simulink model "gm_Transformation_V12"  (R2022a)
settings: Solver=FixedStepDiscrete  StartTime=0.0  StopTime=10.0  RelTol=1e-3
InitFcn:
  | Ts_xadc = 0.1;
undefined symbols (not defined in the file or in its folder): T_25MHz, T_mech
libraries: hdlsllib x14, simulink x13, hdlmdlgenlib x6, simulink_need_slupdate x1
(part 2 of 4)

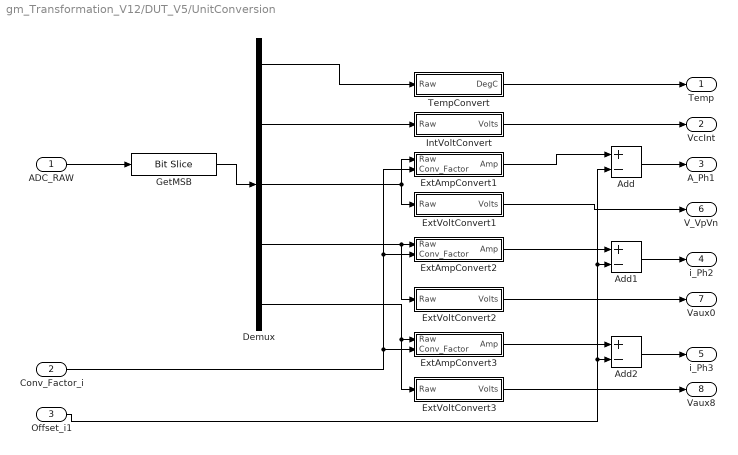
== system gm_Transformation_V12/DUT_V5/UnitConversion ==
  ADC_RAW : Inport
  Conv_Factor_i : Inport  Port=2
  Offset_i1 : Inport  Port=3
  Add : Sum  Inputs=+-  OutDataTypeStr=fixdt(1,16,11)
  Add1 : Sum  Inputs=+-  OutDataTypeStr=fixdt(1,16,11)
  Add2 : Sum  Inputs=+-  OutDataTypeStr=fixdt(1,16,11)
  Demux : Demux  Outputs=5
  ExtAmpConvert1 : Subsystem  TreatAsAtomicUnit=on
  ExtAmpConvert2 : Subsystem  TreatAsAtomicUnit=on
  ExtAmpConvert3 : Subsystem  TreatAsAtomicUnit=on
  ExtVoltConvert1 : Subsystem  TreatAsAtomicUnit=on
  ExtVoltConvert2 : Subsystem  TreatAsAtomicUnit=on
  ExtVoltConvert3 : Subsystem  TreatAsAtomicUnit=on
  GetMSB : hdlsllib/Logic and Bit Operations/Bit Slice  lidx=15  ridx=4
      settings: SourceProductBaseCode=SL
  IntVoltConvert : Subsystem  TreatAsAtomicUnit=on
  TempConvert : Subsystem
  Temp : Outport  VectorParamsAs1DForOutWhenUnconnected=off
  VccInt : Outport  Port=2  VectorParamsAs1DForOutWhenUnconnected=off
  A_Ph1 : Outport  Port=3  VectorParamsAs1DForOutWhenUnconnected=off
  i_Ph2 : Outport  Port=4  VectorParamsAs1DForOutWhenUnconnected=off
  i_Ph3 : Outport  Port=5  VectorParamsAs1DForOutWhenUnconnected=off
  V_VpVn : Outport  Port=6  VectorParamsAs1DForOutWhenUnconnected=off
  Vaux0 : Outport  Port=7  VectorParamsAs1DForOutWhenUnconnected=off
  Vaux8 : Outport  Port=8  VectorParamsAs1DForOutWhenUnconnected=off
  wires:
  Offset_i1/1 -> Add1/2, Add/2, Add2/2
  Add2/1 -> i_Ph3/1
  ExtAmpConvert3/1(Amp) -> Add2/1
  Add1/1 -> i_Ph2/1
  ExtAmpConvert2/1(Amp) -> Add1/1
  Add/1 -> A_Ph1/1
  ExtVoltConvert1/1(Volts) -> V_VpVn/1
  Conv_Factor_i/1 -> ExtAmpConvert1/2(Conv_Factor), ExtAmpConvert2/2(Conv_Factor), ExtAmpConvert3/2(Conv_Factor)
  Demux/5 -> ExtVoltConvert3/1(Raw), ExtAmpConvert3/1(Raw)
  Demux/4 -> ExtAmpConvert2/1(Raw), ExtVoltConvert2/1(Raw)
  Demux/3 -> ExtAmpConvert1/1(Raw), ExtVoltConvert1/1(Raw)
  Demux/2 -> IntVoltConvert/1(Raw)
  Demux/1 -> TempConvert/1(Raw)
  ExtVoltConvert3/1(Volts) -> Vaux8/1
  ExtVoltConvert2/1(Volts) -> Vaux0/1
  ExtAmpConvert1/1(Amp) -> Add/1
  IntVoltConvert/1(Volts) -> VccInt/1
  TempConvert/1(DegC) -> Temp/1
  GetMSB/1 -> Demux/1
  ADC_RAW/1 -> GetMSB/1

== system gm_Transformation_V12/Trans_123_dq_fix_V12/Delay10_controlled ==
  in0 : Inport  OutDataTypeStr=fixdt(1, 18, 11)  SampleTime=4e-08
  stateControl : EnablePort  OutDataTypeStr=boolean
  Delay10 : Delay  DelayLength=double(1)  InitialCondition=0  SampleTime=4e-08
  out0 : Outport  OutDataTypeStr=fixdt(1, 18, 11)  SampleTime=4e-08
  wires:
  Delay10/1 -> out0/1
  in0/1 -> Delay10/1

== system gm_Transformation_V12/Trans_123_dq_fix_V12/Delay16_controlled ==
  in0 : Inport  OutDataTypeStr=fixdt(1, 18, 11)  SampleTime=4e-08
  stateControl : EnablePort  OutDataTypeStr=boolean
  Delay16 : Delay  DelayLength=double(1)  InitialCondition=0  SampleTime=4e-08
  out0 : Outport  OutDataTypeStr=fixdt(1, 18, 11)  SampleTime=4e-08
  wires:
  Delay16/1 -> out0/1
  in0/1 -> Delay16/1

== system gm_Transformation_V12/Trans_123_dq_fix_V12/Delay1_controlled ==
  in0 : Inport  OutDataTypeStr=fixdt(1, 18, 11)  SampleTime=4e-08
  stateControl : EnablePort  OutDataTypeStr=boolean
  Delay1 : Delay  DelayLength=double(1)  InitialCondition=0  SampleTime=4e-08
  out0 : Outport  OutDataTypeStr=fixdt(1, 18, 11)  SampleTime=4e-08
  wires:
  Delay1/1 -> out0/1
  in0/1 -> Delay1/1

== system gm_Transformation_V12/Trans_123_dq_fix_V12/Delay22_controlled ==
  in0 : Inport  OutDataTypeStr=fixdt(1, 18, 11)  SampleTime=4e-08
  stateControl : EnablePort  OutDataTypeStr=boolean
  Delay22 : Delay  DelayLength=double(1)  InitialCondition=0  SampleTime=4e-08
  out0 : Outport  OutDataTypeStr=fixdt(1, 18, 11)  SampleTime=4e-08
  wires:
  Delay22/1 -> out0/1
  in0/1 -> Delay22/1

== system gm_Transformation_V12/Trans_123_dq_fix_V12/Delay2_controlled ==
  in0 : Inport  OutDataTypeStr=fixdt(1, 18, 11)  SampleTime=4e-08
  stateControl : EnablePort  OutDataTypeStr=boolean
  Delay2 : Delay  DelayLength=double(1)  InitialCondition=0  SampleTime=4e-08
  out0 : Outport  OutDataTypeStr=fixdt(1, 18, 11)  SampleTime=4e-08
  wires:
  Delay2/1 -> out0/1
  in0/1 -> Delay2/1

== system gm_Transformation_V12/Trans_123_dq_fix_V12/Delay3_controlled ==
  in0 : Inport  OutDataTypeStr=fixdt(1, 16, 14)  SampleTime=4e-08
  stateControl : EnablePort  OutDataTypeStr=boolean
  Delay3 : Delay  DelayLength=double(1)  InitialCondition=0  SampleTime=4e-08
  out0 : Outport  OutDataTypeStr=fixdt(1, 16, 14)  SampleTime=4e-08
  wires:
  Delay3/1 -> out0/1
  in0/1 -> Delay3/1

== system gm_Transformation_V12/Trans_123_dq_fix_V12/Delay4_controlled ==
  in0 : Inport  OutDataTypeStr=fixdt(1, 18, 11)  SampleTime=4e-08
  stateControl : EnablePort  OutDataTypeStr=boolean
  Delay4 : Delay  DelayLength=double(1)  InitialCondition=0  SampleTime=4e-08
  out0 : Outport  OutDataTypeStr=fixdt(1, 18, 11)  SampleTime=4e-08
  wires:
  Delay4/1 -> out0/1
  in0/1 -> Delay4/1

== system gm_Transformation_V12/Trans_123_dq_fix_V12/Delay5_controlled ==
  in0 : Inport  OutDataTypeStr=fixdt(1, 18, 11)  SampleTime=4e-08
  stateControl : EnablePort  OutDataTypeStr=boolean
  Delay5 : Delay  DelayLength=double(1)  InitialCondition=0  SampleTime=4e-08
  out0 : Outport  OutDataTypeStr=fixdt(1, 18, 11)  SampleTime=4e-08
  wires:
  Delay5/1 -> out0/1
  in0/1 -> Delay5/1

== system gm_Transformation_V12/Trans_123_dq_fix_V12/Delay7_controlled ==
  in0 : Inport  OutDataTypeStr=fixdt(1, 16, 14)  SampleTime=4e-08
  stateControl : EnablePort  OutDataTypeStr=boolean
  Delay7 : Delay  DelayLength=double(1)  InitialCondition=0  SampleTime=4e-08
  out0 : Outport  OutDataTypeStr=fixdt(1, 16, 14)  SampleTime=4e-08
  wires:
  Delay7/1 -> out0/1
  in0/1 -> Delay7/1

== system gm_Transformation_V12/Trans_123_dq_fix_V12/reset_old2_controlled ==
  in0 : Inport  OutDataTypeStr=boolean  SampleTime=4e-08
  stateControl : EnablePort  OutDataTypeStr=boolean
  reset_old2 : Delay  DelayLength=double(1)  InitialCondition=0  SampleTime=4e-08
  out0 : Outport  OutDataTypeStr=boolean  SampleTime=4e-08
  wires:
  reset_old2/1 -> out0/1
  in0/1 -> reset_old2/1

== system gm_Transformation_V12/xadc/xadc_plant ==
  Addr : Inport
  V : Inport  Port=2
  Vaux : Inport  Port=3
  AuxChan : Subsystem
  Bit Slice : hdlsllib/Logic and Bit Operations/Bit Slice  lidx=3  ridx=0
      settings: SourceProductBaseCode=SL
  Bit Slice1 : hdlsllib/Logic and Bit Operations/Bit Slice  lidx=4  ridx=4
      settings: SourceProductBaseCode=SL
  IntChan : Subsystem
  Switch : Switch  Criteria=u2 ~= 0  SaturateOnIntegerOverflow=off  InputSameDT=off
  Data : Outport  VectorParamsAs1DForOutWhenUnconnected=off
  wires:
  AuxChan/1(Aux_ADC) -> Switch/1
  IntChan/1(Int_ADC) -> Switch/3
  Bit Slice1/1 -> Switch/2
  Switch/1 -> Data/1
  V/1 -> IntChan/2(V)
  Vaux/1 -> AuxChan/2(Vaux)
  Bit Slice/1 -> AuxChan/1(Addr), IntChan/1(Addr)
  Addr/1 -> Bit Slice/1, Bit Slice1/1

== system gm_Transformation_V12/DUT_V5/UnitConversion/ExtAmpConvert1 ==
  Raw : Inport
  Conv_Factor : Inport  Port=2
  Product : Product  OutDataTypeStr=fixdt(1,16,11)
  Amp : Outport  VectorParamsAs1DForOutWhenUnconnected=off
  wires:
  Conv_Factor/1 -> Product/2
  Product/1 -> Amp/1
  Raw/1 -> Product/1

== system gm_Transformation_V12/DUT_V5/UnitConversion/ExtAmpConvert2 ==
  Raw : Inport
  Conv_Factor : Inport  Port=2
  Product : Product  OutDataTypeStr=fixdt(1,16,11)
  Amp : Outport  VectorParamsAs1DForOutWhenUnconnected=off
  wires:
  Conv_Factor/1 -> Product/2
  Product/1 -> Amp/1
  Raw/1 -> Product/1

== system gm_Transformation_V12/DUT_V5/UnitConversion/ExtAmpConvert3 ==
  Raw : Inport
  Conv_Factor : Inport  Port=2
  Product : Product  OutDataTypeStr=fixdt(1,16,11)
  Amp : Outport  VectorParamsAs1DForOutWhenUnconnected=off
  wires:
  Conv_Factor/1 -> Product/2
  Product/1 -> Amp/1
  Raw/1 -> Product/1

== system gm_Transformation_V12/DUT_V5/UnitConversion/ExtVoltConvert1 ==
  Raw : Inport
  Gain : Gain  Gain=fi(1/4096)  OutMin=0  OutMax=1  OutDataTypeStr=fixdt(0,16)
  Volts : Outport  VectorParamsAs1DForOutWhenUnconnected=off
  wires:
  Gain/1 -> Volts/1
  Raw/1 -> Gain/1

== system gm_Transformation_V12/DUT_V5/UnitConversion/ExtVoltConvert2 ==
  Raw : Inport
  Gain : Gain  Gain=fi(1/4096)  OutMin=0  OutMax=1  OutDataTypeStr=fixdt(0,16)
  Volts : Outport  VectorParamsAs1DForOutWhenUnconnected=off
  wires:
  Raw/1 -> Gain/1
  Gain/1 -> Volts/1

== system gm_Transformation_V12/DUT_V5/UnitConversion/ExtVoltConvert3 ==
  Raw : Inport
  Gain : Gain  Gain=fi(1/4096)  OutMin=0  OutMax=1  OutDataTypeStr=fixdt(0,16)
  Volts : Outport  VectorParamsAs1DForOutWhenUnconnected=off
  wires:
  Gain/1 -> Volts/1
  Raw/1 -> Gain/1

== system gm_Transformation_V12/DUT_V5/UnitConversion/IntVoltConvert ==
  Raw : Inport
  Gain : Gain  Gain=fi(3/4096)  OutMin=0  OutMax=3  OutDataTypeStr=fixdt(0,16)
  Volts : Outport  VectorParamsAs1DForOutWhenUnconnected=off
  wires:
  Gain/1 -> Volts/1
  Raw/1 -> Gain/1

== system gm_Transformation_V12/DUT_V5/UnitConversion/TempConvert ==
  Raw : Inport
  Add : Sum  Inputs=+-
  Constant : Constant  Value=273.15  OutDataTypeStr=fixdt(0,15)  SampleTime=-1
  Gain : Gain  Gain=fi(503.975/4096)  OutMin=0  OutMax=503.975  OutDataTypeStr=fixdt(0,15)
  DegC : Outport  VectorParamsAs1DForOutWhenUnconnected=off
  wires:
  Raw/1 -> Gain/1
  Add/1 -> DegC/1
  Constant/1 -> Add/2
  Gain/1 -> Add/1

== system gm_Transformation_V12/xadc/xadc_plant/AuxChan ==
  Addr : Inport
  Vaux : Inport  Port=2
  Demux : Demux  Outputs=16
  ExtVoltPlant19 : Subsystem
  Multiport Switch1 : MultiPortSwitch  DataPortOrder=Zero-based contiguous  Inputs=16  DiagnosticForDefault=None  zeroidx=on  SaturateOnIntegerOverflow=off  InputSameDT=off
  Aux_ADC : Outport  VectorParamsAs1DForOutWhenUnconnected=off
  wires:
  Demux/16 -> Multiport Switch1/17
  Addr/1 -> Multiport Switch1/1
  Demux/15 -> Multiport Switch1/16
  Multiport Switch1/1 -> Aux_ADC/1
  Demux/9 -> Multiport Switch1/10
  Vaux/1 -> ExtVoltPlant19/1(Volts)
  Demux/7 -> Multiport Switch1/8
  Demux/5 -> Multiport Switch1/6
  Demux/13 -> Multiport Switch1/14
  Demux/11 -> Multiport Switch1/12
  Demux/10 -> Multiport Switch1/11
  Demux/4 -> Multiport Switch1/5
  Demux/14 -> Multiport Switch1/15
  Demux/6 -> Multiport Switch1/7
  Demux/12 -> Multiport Switch1/13
  Demux/8 -> Multiport Switch1/9
  Demux/2 -> Multiport Switch1/3
  Demux/3 -> Multiport Switch1/4
  Demux/1 -> Multiport Switch1/2
  ExtVoltPlant19/1(Raw_ADC) -> Demux/1

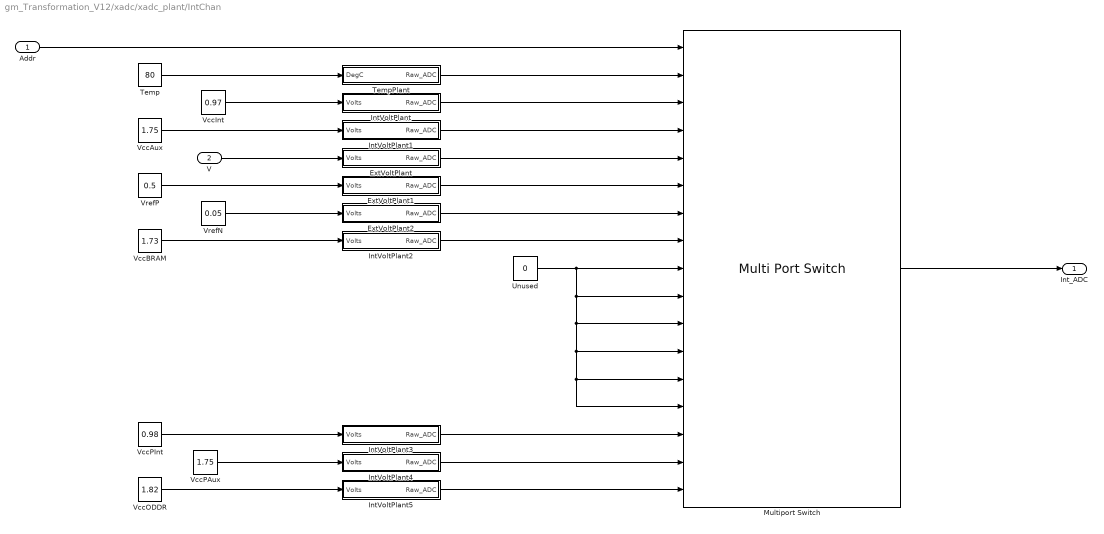
== system gm_Transformation_V12/xadc/xadc_plant/IntChan ==
  Addr : Inport
  V : Inport  Port=2
  ExtVoltPlant : Subsystem
  ExtVoltPlant1 : Subsystem
  ExtVoltPlant2 : Subsystem
  IntVoltPlant : Subsystem
  IntVoltPlant1 : Subsystem
  IntVoltPlant2 : Subsystem
  IntVoltPlant3 : Subsystem
  IntVoltPlant4 : Subsystem
  IntVoltPlant5 : Subsystem
  Multiport Switch : MultiPortSwitch  DataPortOrder=Zero-based contiguous  Inputs=16  DiagnosticForDefault=None  zeroidx=on  SaturateOnIntegerOverflow=off  InputSameDT=off
  Temp : Constant  Value=80  SampleTime=-1
  TempPlant : Subsystem
  Unused : Constant  Value=0  OutDataTypeStr=Inherit: Inherit via back propagation  SampleTime=-1
  VccAux : Constant  Value=1.75  SampleTime=-1
  VccBRAM : Constant  Value=1.73  SampleTime=-1
  VccInt : Constant  Value=0.97  SampleTime=-1
  VccODDR : Constant  Value=1.82  SampleTime=-1
  VccPAux : Constant  Value=1.75  SampleTime=-1
  VccPInt : Constant  Value=0.98  SampleTime=-1
  VrefN : Constant  Value=0.05  SampleTime=-1
  VrefP : Constant  Value=0.5  SampleTime=-1
  Int_ADC : Outport  VectorParamsAs1DForOutWhenUnconnected=off
  wires:
  VrefP/1 -> ExtVoltPlant1/1(Volts)
  ExtVoltPlant1/1(Raw_ADC) -> Multiport Switch/6
  IntVoltPlant1/1(Raw_ADC) -> Multiport Switch/4
  Unused/1 -> Multiport Switch/10, Multiport Switch/11, Multiport Switch/12, Multiport Switch/13, Multiport Switch/14, Multiport Switch/9
  IntVoltPlant/1(Raw_ADC) -> Multiport Switch/3
  Multiport Switch/1 -> Int_ADC/1
  Addr/1 -> Multiport Switch/1
  IntVoltPlant3/1(Raw_ADC) -> Multiport Switch/15
  VccBRAM/1 -> IntVoltPlant2/1(Volts)
  VccAux/1 -> IntVoltPlant1/1(Volts)
  VccPInt/1 -> IntVoltPlant3/1(Volts)
  VccPAux/1 -> IntVoltPlant4/1(Volts)
  ExtVoltPlant/1(Raw_ADC) -> Multiport Switch/5
  Temp/1 -> TempPlant/1(DegC)
  IntVoltPlant4/1(Raw_ADC) -> Multiport Switch/16
  VccInt/1 -> IntVoltPlant/1(Volts)
  TempPlant/1(Raw_ADC) -> Multiport Switch/2
  ExtVoltPlant2/1(Raw_ADC) -> Multiport Switch/7
  V/1 -> ExtVoltPlant/1(Volts)
  IntVoltPlant5/1(Raw_ADC) -> Multiport Switch/17
  VrefN/1 -> ExtVoltPlant2/1(Volts)
  VccODDR/1 -> IntVoltPlant5/1(Volts)
  IntVoltPlant2/1(Raw_ADC) -> Multiport Switch/8

== system gm_Transformation_V12/xadc/xadc_plant/AuxChan/ExtVoltPlant19 ==
  Volts : Inport
  Bit Concat : hdlsllib/Logic and Bit Operations/Bit Concat  numInputs=2
  Data Type Conversion : DataTypeConversion  OutDataTypeStr=fixdt(0,12,0)  SaturateOnIntegerOverflow=off  RndMeth=Floor
  Gain : Gain  Gain=4096
  LSB : Constant  Value=fi(0,0,4,0)  SampleTime=-1
  Raw_ADC : Outport  VectorParamsAs1DForOutWhenUnconnected=off
  wires:
  Gain/1 -> Data Type Conversion/1
  Volts/1 -> Gain/1
  Data Type Conversion/1 -> Bit Concat/1
  LSB/1 -> Bit Concat/2
  Bit Concat/1 -> Raw_ADC/1

== system gm_Transformation_V12/xadc/xadc_plant/IntChan/ExtVoltPlant ==
  Volts : Inport
  Bit Concat : hdlsllib/Logic and Bit Operations/Bit Concat  numInputs=2
  Data Type Conversion : DataTypeConversion  OutDataTypeStr=fixdt(0,12,0)  SaturateOnIntegerOverflow=off  RndMeth=Floor
  Gain : Gain  Gain=4096
  LSB : Constant  Value=fi(0,0,4,0)  SampleTime=-1
  Raw_ADC : Outport  VectorParamsAs1DForOutWhenUnconnected=off
  wires:
  Gain/1 -> Data Type Conversion/1
  Volts/1 -> Gain/1
  Data Type Conversion/1 -> Bit Concat/1
  LSB/1 -> Bit Concat/2
  Bit Concat/1 -> Raw_ADC/1

== system gm_Transformation_V12/xadc/xadc_plant/IntChan/ExtVoltPlant1 ==
  Volts : Inport
  Bit Concat : hdlsllib/Logic and Bit Operations/Bit Concat  numInputs=2
  Data Type Conversion : DataTypeConversion  OutDataTypeStr=fixdt(0,12,0)  SaturateOnIntegerOverflow=off  RndMeth=Floor
  Gain : Gain  Gain=4096
  LSB : Constant  Value=fi(0,0,4,0)  SampleTime=-1
  Raw_ADC : Outport  VectorParamsAs1DForOutWhenUnconnected=off
  wires:
  Bit Concat/1 -> Raw_ADC/1
  LSB/1 -> Bit Concat/2
  Data Type Conversion/1 -> Bit Concat/1
  Volts/1 -> Gain/1
  Gain/1 -> Data Type Conversion/1

== system gm_Transformation_V12/xadc/xadc_plant/IntChan/ExtVoltPlant2 ==
  Volts : Inport
  Bit Concat : hdlsllib/Logic and Bit Operations/Bit Concat  numInputs=2
  Data Type Conversion : DataTypeConversion  OutDataTypeStr=fixdt(0,12,0)  SaturateOnIntegerOverflow=off  RndMeth=Floor
  Gain : Gain  Gain=4096
  LSB : Constant  Value=fi(0,0,4,0)  SampleTime=-1
  Raw_ADC : Outport  VectorParamsAs1DForOutWhenUnconnected=off
  wires:
  Gain/1 -> Data Type Conversion/1
  Volts/1 -> Gain/1
  Data Type Conversion/1 -> Bit Concat/1
  LSB/1 -> Bit Concat/2
  Bit Concat/1 -> Raw_ADC/1

== system gm_Transformation_V12/xadc/xadc_plant/IntChan/IntVoltPlant ==
  Volts : Inport
  Bit Concat : hdlsllib/Logic and Bit Operations/Bit Concat  numInputs=2
  Data Type Conversion : DataTypeConversion  OutDataTypeStr=fixdt(0,12,0)  SaturateOnIntegerOverflow=off  RndMeth=Floor
  Gain : Gain  Gain=4096/3
  LSB : Constant  Value=fi(0,0,4,0)  SampleTime=-1
  Raw_ADC : Outport  VectorParamsAs1DForOutWhenUnconnected=off
  wires:
  Bit Concat/1 -> Raw_ADC/1
  LSB/1 -> Bit Concat/2
  Data Type Conversion/1 -> Bit Concat/1
  Volts/1 -> Gain/1
  Gain/1 -> Data Type Conversion/1

== system gm_Transformation_V12/xadc/xadc_plant/IntChan/IntVoltPlant1 ==
  Volts : Inport
  Bit Concat : hdlsllib/Logic and Bit Operations/Bit Concat  numInputs=2
  Data Type Conversion : DataTypeConversion  OutDataTypeStr=fixdt(0,12,0)  SaturateOnIntegerOverflow=off  RndMeth=Floor
  Gain : Gain  Gain=4096/3
  LSB : Constant  Value=fi(0,0,4,0)  SampleTime=-1
  Raw_ADC : Outport  VectorParamsAs1DForOutWhenUnconnected=off
  wires:
  Gain/1 -> Data Type Conversion/1
  Volts/1 -> Gain/1
  Data Type Conversion/1 -> Bit Concat/1
  LSB/1 -> Bit Concat/2
  Bit Concat/1 -> Raw_ADC/1

== system gm_Transformation_V12/xadc/xadc_plant/IntChan/IntVoltPlant2 ==
  Volts : Inport
  Bit Concat : hdlsllib/Logic and Bit Operations/Bit Concat  numInputs=2
  Data Type Conversion : DataTypeConversion  OutDataTypeStr=fixdt(0,12,0)  SaturateOnIntegerOverflow=off  RndMeth=Floor
  Gain : Gain  Gain=4096/3
  LSB : Constant  Value=fi(0,0,4,0)  SampleTime=-1
  Raw_ADC : Outport  VectorParamsAs1DForOutWhenUnconnected=off
  wires:
  Bit Concat/1 -> Raw_ADC/1
  LSB/1 -> Bit Concat/2
  Data Type Conversion/1 -> Bit Concat/1
  Volts/1 -> Gain/1
  Gain/1 -> Data Type Conversion/1

== system gm_Transformation_V12/xadc/xadc_plant/IntChan/IntVoltPlant3 ==
  Volts : Inport
  Bit Concat : hdlsllib/Logic and Bit Operations/Bit Concat  numInputs=2
  Data Type Conversion : DataTypeConversion  OutDataTypeStr=fixdt(0,12,0)  SaturateOnIntegerOverflow=off  RndMeth=Floor
  Gain : Gain  Gain=4096/3
  LSB : Constant  Value=fi(0,0,4,0)  SampleTime=-1
  Raw_ADC : Outport  VectorParamsAs1DForOutWhenUnconnected=off
  wires:
  Gain/1 -> Data Type Conversion/1
  Volts/1 -> Gain/1
  Data Type Conversion/1 -> Bit Concat/1
  LSB/1 -> Bit Concat/2
  Bit Concat/1 -> Raw_ADC/1

== system gm_Transformation_V12/xadc/xadc_plant/IntChan/IntVoltPlant4 ==
  Volts : Inport
  Bit Concat : hdlsllib/Logic and Bit Operations/Bit Concat  numInputs=2
  Data Type Conversion : DataTypeConversion  OutDataTypeStr=fixdt(0,12,0)  SaturateOnIntegerOverflow=off  RndMeth=Floor
  Gain : Gain  Gain=4096/3
  LSB : Constant  Value=fi(0,0,4,0)  SampleTime=-1
  Raw_ADC : Outport  VectorParamsAs1DForOutWhenUnconnected=off
  wires:
  Bit Concat/1 -> Raw_ADC/1
  LSB/1 -> Bit Concat/2
  Data Type Conversion/1 -> Bit Concat/1
  Volts/1 -> Gain/1
  Gain/1 -> Data Type Conversion/1

== system gm_Transformation_V12/xadc/xadc_plant/IntChan/IntVoltPlant5 ==
  Volts : Inport
  Bit Concat : hdlsllib/Logic and Bit Operations/Bit Concat  numInputs=2
  Data Type Conversion : DataTypeConversion  OutDataTypeStr=fixdt(0,12,0)  SaturateOnIntegerOverflow=off  RndMeth=Floor
  Gain : Gain  Gain=4096/3
  LSB : Constant  Value=fi(0,0,4,0)  SampleTime=-1
  Raw_ADC : Outport  VectorParamsAs1DForOutWhenUnconnected=off
  wires:
  Gain/1 -> Data Type Conversion/1
  Volts/1 -> Gain/1
  Data Type Conversion/1 -> Bit Concat/1
  LSB/1 -> Bit Concat/2
  Bit Concat/1 -> Raw_ADC/1

== system gm_Transformation_V12/xadc/xadc_plant/IntChan/TempPlant ==
  DegC : Inport
  Add : Sum
  Bit Concat : hdlsllib/Logic and Bit Operations/Bit Concat  numInputs=2
  Data Type Conversion : DataTypeConversion  OutDataTypeStr=fixdt(0,12,0)  SaturateOnIntegerOverflow=off  RndMeth=Floor
  Gain : Gain  Gain=4096/503.975
  LSB : Constant  Value=fi(0,0,4,0)  SampleTime=-1
  Offset : Constant  Value=273.15  SampleTime=-1
  Raw_ADC : Outport  VectorParamsAs1DForOutWhenUnconnected=off
  wires:
  Bit Concat/1 -> Raw_ADC/1
  Gain/1 -> Data Type Conversion/1
  LSB/1 -> Bit Concat/2
  Data Type Conversion/1 -> Bit Concat/1
  Add/1 -> Gain/1
  DegC/1 -> Add/1
  Offset/1 -> Add/2

== matlab function gm_Transformation_V12/Trans_123_dq_fix_V3/dq_transformation ==
  data: a input; d output; b input; theta input; q output
% Author : Saeid Saeidi
% Modified: Sebastian Wendel
% EAL -TUM
% MATLAB Version : R2016a
function [d, q]= fcn(a,b, theta )
% Defining persistent variables
%In VHDL , persistent variables will appear as Signals
persistent i1
persistent i2
persistent i3
persistent i4
persistent i5
persistent i6
persistent i7
persistent i8
persistent i9
persistent i10
persistent i11
persistent i12
persistent i13
persistent i14
persistent i15
persistent i16
% %
persistent i1n
persistent i2n
persistent i3n
persistent i4n
persistent i5n
persistent i6n
persistent i7n
persistent i8n
persistent i9n
persistent i10n
persistent i11n
persistent i12n
persistent i13n
persistent i14n
persistent i15n
persistent i16n
% %
persistent a1
persistent a2
persistent a3
persistent a4
persistent a5
persistent a6
persistent a7
persistent a8
persistent a9
persistent a10
persistent a11
persistent a12
persistent a13
persistent a14
persistent a15
persistent a16
% %
persistent b1
persistent b2
persistent b3
persistent b4
persistent b5
persistent b6
persistent b7
persistent b8
persistent b9
persistent b10
persistent b11
persistent b12
persistent b13
persistent b14
persistent b15
persistent b16
% %
persistent beta1
persistent beta2
persistent beta3
persistent beta4
persistent beta5
persistent beta6
persistent beta7
persistent beta8
persistent beta9
persistent beta10
persistent beta11
persistent beta12
persistent beta13
persistent beta14
persistent beta15
% %
persistent a1n
persistent a2n
persistent a3n
persistent a4n
persistent a5n
persistent a6n
persistent a7n
persistent a8n
persistent a9n
persistent a10n
persistent a11n
persistent a12n
persistent a13n
persistent a14n
persistent a15n
persistent a16n
% %
persistent b1n
persistent b2n
persistent b3n
persistent b4n
persistent b5n
persistent b6n
persistent b7n
persistent b8n
persistent b9n
persistent b10n
persistent b11n
persistent b12n
persistent b13n
persistent b14n
persistent b15n
persistent b16n
% %
persistent beta1n
persistent beta2n
persistent beta3n
persistent beta4n
persistent beta5n
persistent beta6n
persistent beta7n
persistent beta8n
persistent beta9n
persistent beta10n
persistent beta11n
persistent beta12n
persistent beta13n
persistent beta14n
persistent beta15n
% %
% Initialization of Persistent Variables with the numeric type of the
% input variables "a" and "b"
% After generating VHDL this part will be located in the RESET
if isempty (a1)
a1 = fi (0, numerictype (a), hdlfimath );
a2 = fi (0, numerictype (a), hdlfimath );
a3 = fi (0, numerictype (a), hdlfimath );
a4 = fi (0, numerictype (a), hdlfimath );
a5 = fi (0, numerictype (a), hdlfimath );
a6 = fi (0, numerictype (a), hdlfimath );
a7 = fi (0, numerictype (a), hdlfimath );
a8 = fi (0, numerictype (a), hdlfimath );
a9 = fi (0, numerictype (a), hdlfimath );
a10 = fi (0, numerictype (a), hdlfimath );
a11 = fi (0, numerictype (a), hdlfimath );
a12 = fi (0, numerictype (a), hdlfimath );
a13 = fi (0, numerictype (a), hdlfimath );
a14 = fi (0, numerictype (a), hdlfimath );
a15 = fi (0, numerictype (a), hdlfimath );
a16 = fi (0, numerictype (a), hdlfimath );
% %
b1 = fi (0, numerictype (b), hdlfimath );
b2 = fi (0, numerictype (b), hdlfimath );
b3 = fi (0, numerictype (b), hdlfimath );
b4 = fi (0, numerictype (b), hdlfimath );
b5 = fi (0, numerictype (b), hdlfimath );
b6 = fi (0, numerictype (b), hdlfimath );
b7 = fi (0, numerictype (b), hdlfimath );
b8 = fi (0, numerictype (b), hdlfimath );
b9 = fi (0, numerictype (b), hdlfimath );
b10 = fi (0, numerictype (b), hdlfimath );
b11 = fi (0, numerictype (b), hdlfimath );
b12 = fi (0, numerictype (b), hdlfimath );
b13 = fi (0, numerictype (b), hdlfimath );
b14 = fi (0, numerictype (b), hdlfimath );
b15 = fi (0, numerictype (b), hdlfimath );
b16 = fi (0, numerictype (b), hdlfimath );
% %
beta1 = fi (0, numerictype ( theta ), hdlfimath );
beta2 = fi (0, numerictype ( theta ), hdlfimath );
beta3 = fi (0, numerictype ( theta ), hdlfimath );
beta4 = fi (0, numerictype ( theta ), hdlfimath );
beta5 = fi (0, numerictype ( theta ), hdlfimath );
beta6 = fi (0, numerictype ( theta ), hdlfimath );
beta7 = fi (0, numerictype ( theta ), hdlfimath );
beta8 = fi (0, numerictype ( theta ), hdlfimath );
beta9 = fi (0, numerictype ( theta ), hdlfimath );
beta10 = fi (0, numerictype ( theta ), hdlfimath );
beta11 = fi (0, numerictype ( theta ), hdlfimath );
beta12 = fi (0, numerictype ( theta ), hdlfimath );
beta13 = fi (0, numerictype ( theta ), hdlfimath );
beta14 = fi (0, numerictype ( theta ), hdlfimath );
beta15 = fi (0, numerictype ( theta ), hdlfimath );
% %
a1n = fi (0, numerictype (a), hdlfimath );
a2n = fi (0, numerictype (a), hdlfimath );
a3n = fi (0, numerictype (a), hdlfimath );
a4n = fi (0, numerictype (a), hdlfimath );
a5n = fi (0, numerictype (a), hdlfimath );
a6n = fi (0, numerictype (a), hdlfimath );
a7n = fi (0, numerictype (a), hdlfimath );
a8n = fi (0, numerictype (a), hdlfimath );
a9n = fi (0, numerictype (a), hdlfimath );
a10n = fi (0, numerictype (a), hdlfimath );
a11n = fi (0, numerictype (a), hdlfimath );
a12n = fi (0, numerictype (a), hdlfimath );
a13n = fi (0, numerictype (a), hdlfimath );
a14n = fi (0, numerictype (a), hdlfimath );
a15n = fi (0, numerictype (a), hdlfimath );
a16n = fi (0, numerictype (a), hdlfimath );
% %
b1n = fi (0, numerictype (b), hdlfimath );
b2n = fi (0, numerictype (b), hdlfimath );
b3n = fi (0, numerictype (b), hdlfimath );
b4n = fi (0, numerictype (b), hdlfimath );
b5n = fi (0, numerictype (b), hdlfimath );
b6n = fi (0, numerictype (b), hdlfimath );
b7n = fi (0, numerictype (b), hdlfimath );
b8n = fi (0, numerictype (b), hdlfimath );
b9n = fi (0, numerictype (b), hdlfimath );
b10n = fi (0, numerictype (b), hdlfimath );
b11n = fi (0, numerictype (b), hdlfimath );
b12n = fi (0, numerictype (b), hdlfimath );
b13n = fi (0, numerictype (b), hdlfimath );
b14n = fi (0, numerictype (b), hdlfimath );
b15n = fi (0, numerictype (b), hdlfimath );
b16n = fi (0, numerictype (b), hdlfimath );
% %
beta1n = fi (0, numerictype ( theta ), hdlfimath );
beta2n = fi (0, numerictype ( theta ), hdlfimath );
beta3n = fi (0, numerictype ( theta ), hdlfimath );
beta4n = fi (0, numerictype ( theta ), hdlfimath );
beta5n = fi (0, numerictype ( theta ), hdlfimath );
beta6n = fi (0, numerictype ( theta ), hdlfimath );
beta7n = fi (0, numerictype ( theta ), hdlfimath );
beta8n = fi (0, numerictype ( theta ), hdlfimath );
beta9n = fi (0, numerictype ( theta ), hdlfimath );
beta10n = fi (0, numerictype ( theta ), hdlfimath );
beta11n = fi (0, numerictype ( theta ), hdlfimath );
beta12n = fi (0, numerictype ( theta ), hdlfimath );
beta13n = fi (0, numerictype ( theta ), hdlfimath );
beta14n = fi (0, numerictype ( theta ), hdlfimath );
beta15n = fi (0, numerictype ( theta ), hdlfimath );
% %
i1n = ufi (0 ,1 ,0);
i2n = ufi (0 ,1 ,0);
i3n = ufi (0 ,1 ,0);
i4n = ufi (0 ,1 ,0);
i5n = ufi (0 ,1 ,0);
i6n = ufi (0 ,1 ,0);
i7n = ufi (0 ,1 ,0);
i8n = ufi (0 ,1 ,0);
i9n = ufi (0 ,1 ,0);
i10n = ufi (0 ,1 ,0);
i11n = ufi (0 ,1 ,0);
i12n = ufi (0 ,1 ,0);
i13n = ufi (0 ,1 ,0);
i14n = ufi (0 ,1 ,0);
i15n = ufi (0 ,1 ,0);
i16n = ufi (0 ,1 ,0);
% %
i1 = ufi (0 ,1 ,0);
i2 = ufi (0 ,1 ,0);
i3 = ufi (0 ,1 ,0);
i4 = ufi (0 ,1 ,0);
i5 = ufi (0 ,1 ,0);
i6 = ufi (0 ,1 ,0);
i7 = ufi (0 ,1 ,0);
i8 = ufi (0 ,1 ,0);
i9 = ufi (0 ,1 ,0);
i10 = ufi (0 ,1 ,0);
i11 = ufi (0 ,1 ,0);
i12 = ufi (0 ,1 ,0);
i13 = ufi (0 ,1 ,0);
i14 = ufi (0 ,1 ,0);
i15 = ufi (0 ,1 ,0);
i16 = ufi (0 ,1 ,0);
end
%-----------------------------------------------------------------------%

% Definition of Constant Values
p       = fi(pi , numerictype ( theta ), hdlfimath );
p2      = fi(pi /2, numerictype ( theta ), hdlfimath ); %1.570796
p2m     = fi(-pi /2, numerictype ( theta ), hdlfimath );
theta0  = fi(theta , numerictype ( theta ), hdlfimath );

% Determining section of the theta -> Check if theta is between -pi/2 and
% pi/2
% -- ------- # First pipeline stage
if( theta0 <= fi(p2m , numerictype ( theta ), hdlfimath ))
    beta1n = fi( theta0 + p, numerictype ( theta ), hdlfimath );
    i1n = ufi (0 ,1 ,0);
elseif ( theta0 >= fi(p2 , numerictype ( theta ), hdlfimath ))
    beta1n = fi( theta0 - p, numerictype ( theta ), hdlfimath );
    i1n = ufi (0 ,1 ,0);
else
    beta1n = theta0 ;
    i1n = ufi (1 ,1 ,0);
end
a1n = fi(a, numerictype (a), hdlfimath );
b1n = fi(b, numerictype (b), hdlfimath );

% -- ------- # Second pipeline stage 0.78539816339745 = pi/4
if( beta1 <fi (0, numerictype ( theta ), hdlfimath ))
    a2n = fi(a1 + b1 , numerictype (a), hdlfimath );
    b2n = fi(b1 - a1 , numerictype (b), hdlfimath );
    beta2n = fi( beta1 + fi (0.78539816339745 , numerictype ( theta ) ,...
    hdlfimath ), numerictype ( theta ), hdlfimath );
else
    a2n = fi(a1 - b1 , numerictype (a), hdlfimath );
    b2n = fi(b1 + a1 , numerictype (b), hdlfimath );
    beta2n = fi( beta1 - fi (0.78539816339745 , numerictype ( theta ) ,...
    hdlfimath ), numerictype ( theta ), hdlfimath );
end

% -- ------- # Third pipeline stage 0.46364760900081 = pi/8 ???
if(beta2 <fi (0, numerictype ( theta ), hdlfimath ))
    a3n = fi(a2 + bitsra (b2 ,1) , numerictype (b), hdlfimath );
    b3n = fi(b2 - bitsra (a2 ,1) , numerictype (a), hdlfimath );
    beta3n = fi( beta2 + fi (0.46364760900081 , numerictype ( theta ) ,...
    hdlfimath ), numerictype ( theta ), hdlfimath );
else
    a3n = fi(a2 - bitsra (b2 ,1) , numerictype (a), hdlfimath );
    b3n = fi(b2 + bitsra (a2 ,1) , numerictype (b), hdlfimath );
    beta3n = fi( beta2 - fi (0.46364760900081 , numerictype ( theta ) ,...
    hdlfimath ), numerictype ( theta ), hdlfimath );
end

% -- ------- # Fourth pipeline stage
if(beta3 <fi (0, numerictype ( theta ), hdlfimath ))
    a4n = fi(a3 + bitsra (b3 ,2) , numerictype (a), hdlfimath );
    b4n = fi(b3 - bitsra (a3 ,2) , numerictype (b), hdlfimath );
    beta4n = fi( beta3 + fi (0.24497866312686 , numerictype ( theta ) ,...
    hdlfimath ), numerictype ( theta ), hdlfimath );
else
    a4n = fi(a3 - bitsra (b3 ,2) , numerictype (a), hdlfimath );
    b4n = fi(b3 + bitsra (a3 ,2) , numerictype (b), hdlfimath );
    beta4n = fi( beta3 - fi (0.24497866312686 , numerictype ( theta ) ,...
    hdlfimath ), numerictype ( theta ), hdlfimath );
end

% -- ------- # Fifth pipeline stage
if(beta4 <fi (0, numerictype ( theta ), hdlfimath ))
    a5n = fi(a4 + bitsra (b4 ,3) , numerictype (a), hdlfimath );
    b5n = fi(b4 - bitsra (a4 ,3) , numerictype (b), hdlfimath );
    beta5n = fi( beta4 + fi (0.12435499454676 , numerictype ( theta ) ,...
    hdlfimath ), numerictype ( theta ), hdlfimath );
else
    a5n = fi(a4 - bitsra (b4 ,3) , numerictype (a), hdlfimath );
    b5n = fi(b4 + bitsra (a4 ,3) , numerictype (b), hdlfimath );
    beta5n = fi( beta4 - fi (0.12435499454676 , numerictype ( theta ) ,...
    hdlfimath ), numerictype ( theta ), hdlfimath );
end

% -- ------- # Sixth pipeline stage
if(beta5 <fi (0, numerictype ( theta ), hdlfimath ))
    a6n = fi(a5 + bitsra (b5 ,4) , numerictype (a), hdlfimath );
    b6n = fi(b5 - bitsra (a5 ,4) , numerictype (b), hdlfimath );
    beta6n = fi( beta5 + fi (0.06241880999596 , numerictype ( theta ) ,...
    hdlfimath ), numerictype ( theta ), hdlfimath );
else
    a6n = fi(a5 - bitsra (b5 ,4) , numerictype (a), hdlfimath );
    b6n = fi( b5 + bitsra (a5 ,4) , numerictype (b), hdlfimath );
    beta6n = fi( beta5 - fi (0.06241880999596 , numerictype ( theta ) ,...
    hdlfimath ), numerictype ( theta ), hdlfimath );
end

% -- ------- # Seventh pipeline stage
if(beta6 <fi (0, numerictype ( theta ), hdlfimath ))
    a7n = fi(a6 + bitsra (b6 ,5) , numerictype (a), hdlfimath );
    b7n = fi(b6 - bitsra (a6 ,5) , numerictype (b), hdlfimath );
    beta7n = fi( beta6 + fi (0.03123983343027 , numerictype ( theta ) ,...
    hdlfimath ), numerictype ( theta ), hdlfimath );
else
    a7n = fi(a6 - bitsra (b6 ,5) , numerictype (a), hdlfimath );
    b7n = fi(b6 + bitsra (a6 ,5) , numerictype (b), hdlfimath );
    beta7n = fi( beta6 - fi (0.03123983343027 , numerictype ( theta ) ,...
    hdlfimath ), numerictype ( theta ), hdlfimath );
end

% -- ------- # Eighth pipeline stage
if(beta7 <fi (0, numerictype ( theta ), hdlfimath ))
    a8n = fi(a7 + bitsra (b7 ,6) , numerictype (a), hdlfimath );
    b8n = fi(b7 - bitsra (a7 ,6) , numerictype (b), hdlfimath );
    beta8n = fi( beta7 + fi (0.01562372862048 , numerictype ( theta ) ,...
    hdlfimath ), numerictype ( theta ), hdlfimath );
else
    a8n = fi(a7 - bitsra (b7 ,6) , numerictype (a), hdlfimath );
    b8n = fi(b7 + bitsra (a7 ,6) , numerictype (b), hdlfimath );
    beta8n = fi( beta7 - fi (0.01562372862048 , numerictype ( theta ) ,...
    hdlfimath ), numerictype ( theta ), hdlfimath );
end

% -- ------- # Ninth pipeline stage
if(beta8 <fi (0, numerictype ( theta ), hdlfimath ))
    a9n = fi(a8 + bitsra (b8 ,7) , numerictype (a), hdlfimath );
    b9n = fi(b8 - bitsra (a8 ,7) , numerictype (b), hdlfimath );
    beta9n = fi( beta8 + fi( 0.00781234106010 , numerictype ( theta ) ,...
    hdlfimath ), numerictype ( theta ), hdlfimath );
else
    a9n = fi(a8 - bitsra (b8 ,7) , numerictype (a), hdlfimath );
    b9n = fi( b8 + bitsra (a8 ,7) , numerictype (b), hdlfimath );
    beta9n = fi( beta8 - fi( 0.00781234106010 , numerictype ( theta ) ,...
    hdlfimath ), numerictype ( theta ), hdlfimath );
end

% -- ------- # Tenth pipeline stage
if(beta9 <fi (0, numerictype ( theta ), hdlfimath ))
    a10n = fi(a9 + bitsra (b9 ,8) , numerictype (a), hdlfimath );
    b10n = fi(b9 - bitsra (a9 ,8) , numerictype (b), hdlfimath );
    beta10n = fi( beta9 + fi (0.00390623013197 , numerictype ( theta ) ,...
    hdlfimath ), numerictype ( theta ), hdlfimath );
else
    a10n = fi(a9 - bitsra (b9 ,8) , numerictype (a), hdlfimath );
    b10n = fi(b9 + bitsra (a9 ,8) , numerictype (b), hdlfimath );
    beta10n = fi( beta9 - fi (0.00390623013197 , numerictype ( theta ) ,...
    hdlfimath ), numerictype ( theta ), hdlfimath );
end

% -- ------- # Eleventh pipeline stage
if( beta10 <fi (0, numerictype ( theta ), hdlfimath ))
    a11n = fi(a10 + bitsra (b10 ,9) , numerictype (a), hdlfimath );
    b11n = fi(b10 - bitsra (a10 ,9) , numerictype (b), hdlfimath );
    beta11n = fi( beta10 + fi (0.00195312251648 , numerictype ( theta ) ,...
    hdlfimath ), numerictype ( theta ), hdlfimath );
else
    a11n = fi(a10 - bitsra (b10 ,9) , numerictype (a), hdlfimath );
    b11n = fi(b10 + bitsra (a10 ,9) , numerictype (b), hdlfimath );
    beta11n = fi( beta10 - fi (0.00195312251648 , numerictype ( theta ) ,...
    hdlfimath ), numerictype ( theta ), hdlfimath );
end

% -- ------- # Twelfth pipeline stage
if( beta11 <fi (0, numerictype ( theta ), hdlfimath ))
    a12n = fi( a11 + bitsra (b11 ,10) , numerictype (a), hdlfimath );
    b12n = fi(b11 - bitsra (a11 ,10) , numerictype (b), hdlfimath );
    beta12n = fi( beta11 + fi (0.00097656218956 , numerictype ( theta ) ,...
    hdlfimath ), numerictype ( theta ), hdlfimath );
else
    a12n = fi(a11 - bitsra (b11 ,10) , numerictype (a), hdlfimath );
    b12n = fi( b11 + bitsra (a11 ,10) , numerictype (b), hdlfimath );
    beta12n = fi( beta11 - fi (0.00097656218956 , numerictype ( theta ) ,...
    hdlfimath ), numerictype ( theta ), hdlfimath );
end

% -- ------- # Thirteenth pipeline stage
if( beta12 <fi (0, numerictype ( theta ), hdlfimath ))
    a13n = fi( a12 + bitsra (b12 ,11) , numerictype (a), hdlfimath );
    b13n = fi(b12 - bitsra (a12 ,11) , numerictype (b), hdlfimath );
    beta13n = fi( beta12 + fi (0.00048828121119 ,numerictype ( theta ) ,...
    hdlfimath ), numerictype ( theta ), hdlfimath );
else
    a13n = fi(a12 - bitsra (b12 ,11) , numerictype (a), hdlfimath );
    b13n = fi( b12 + bitsra (a12 ,11) , numerictype (b), hdlfimath );
    beta13n = fi( beta12 - fi (0.00048828121119 ,numerictype ( theta ) ,...
    hdlfimath ), numerictype ( theta ), hdlfimath );
end

% -- ------- # Fourteenth pipeline stage
if( beta13 <fi (0, numerictype ( theta ), hdlfimath ))
    a14n = fi( a13 + bitsra (b13 ,12) , numerictype (a), hdlfimath );
    b14n = fi(b13 - bitsra (a13 ,12) , numerictype (b), hdlfimath );
    beta14n = fi( beta13 + fi( 0.00024414062015 , numerictype ( theta ) ,...
    hdlfimath ), numerictype ( theta ), hdlfimath );
else
    a14n = fi(a13 - bitsra (b13 ,12) , numerictype (a), hdlfimath );
    b14n = fi( b13 + bitsra (a13 ,12) , numerictype (b), hdlfimath );
    beta14n = fi( beta11 - fi( 0.00024414062015 , numerictype ( theta ) ,...
    hdlfimath ), numerictype ( theta ), hdlfimath );
end

% -- ------- # Fifteenth pipeline stage
if( beta14 <fi (0, numerictype ( theta ), hdlfimath ))
    a15n = fi( a14 + bitsra (b14 ,13) , numerictype (a), hdlfimath );
    b15n = fi(b14 - bitsra (a14 ,13) , numerictype (b), hdlfimath );
    beta15n = fi( beta14 + fi (0.00012207031189 , numerictype ( theta ) ,...
    hdlfimath ), numerictype ( theta ), hdlfimath );
else
    a15n = fi(a14 - bitsra (b14 ,13) , numerictype (a), hdlfimath );
    b15n = fi( b14 + bitsra (a14 ,13) , numerictype (b), hdlfimath );
    beta15n = fi( beta14 - fi (0.00012207031189 , numerictype ( theta ) ,...
    hdlfimath ), numerictype ( theta ), hdlfimath );
end

% -- ------- # Sixteenth pipeline stage
a16n = fi(a15 * sfi ( 0.60725293538591 ,18 ,17) , numerictype (a), hdlfimath );
b16n = fi(b15 * sfi ( 0.60725293538591 ,18 ,17) , numerictype (b), hdlfimath );

% Output Update of Registers
i2n = i1;
i3n = i2;
i4n = i3;
i5n = i4;
i6n = i5;
i7n = i6;
i8n = i7;
i9n = i8;
i10n = i9;
i11n = i10 ;
i12n = i11 ;
i13n = i12 ;
i14n = i13 ;
i15n = i14 ;
i16n = i15 ;
% %
a1 = a1n;
a2 = a2n;
a3 = a3n;
a4 = a4n;
a5 = a5n;
a6 = a6n;
a7 = a7n;
a8 = a8n;
a9 = a9n;
a10 = a10n ;
a11 = a11n ;
a12 = a12n ;
a13 = a13n ;
a14 = a14n ;
a15 = a15n ;
a16 = a16n ;
% %
b1 = b1n;
b2 = b2n;
b3 = b3n;
b4 = b4n;
b5 = b5n;
b6 = b6n;
b7 = b7n;
b8 = b8n;
b9 = b9n;
b10 = b10n ;

b11 = b11n ;
b12 = b12n ;
b13 = b13n ;
b14 = b14n ;
b15 = b15n ;
b16 = b16n ;
% %
beta1 = beta1n ;
beta2 = beta2n ;
beta3 = beta3n ;
beta4 = beta4n ;
beta5 = beta5n ;
beta6 = beta6n ;
beta7 = beta7n ;
beta8 = beta8n ;
beta9 = beta9n ;
beta10 = beta10n ;
beta11 = beta11n ;
beta12 = beta12n ;
beta13 = beta13n ;
beta14 = beta14n ;
beta15 = beta15n ;
% %
i1 = i1n;
i2 = i2n;
i3 = i3n;
i4 = i4n;
i5 = i5n;
i6 = i6n;
i7 = i7n;
i8 = i8n;
i9 = i9n;
i10 = i10n ;
i11 = i11n ;
i12 = i12n ;
i13 = i13n ;
i14 = i14n ;
i15 = i15n ;
i16 = i16n ;
% %
% Generating output
if( i16 == ufi (0 ,1 ,0))
d = -a16;
q = -b16;
else
d = a16;
q = b16;
end

== matlab function gm_Transformation_V12/DUT_V5/xadc_ctrl ==
  data: den_o output; drdy_i input; daddr_o output; do_i input; val_o output
function [den_o, daddr_o, val_o] = xadc_ctrl(drdy_i, do_i)
%#codegen

%% Constants and defines
% Fixed point data types
FM = hdlfimath;
NT_ADDR = numerictype(false,7,0); % Address
NT_VAL = numerictype(false,16,0); % Value
NT_STATE = numerictype(false,2,0); % State

% The state machine will loop over the defined addresses
% reading out each value
% See Xilinx ug480 for more information
ADDR_SEQ = fi([0 1 3 16 24], ... % Value addresses
               NT_ADDR,FM);

NUM_VALS = numel(ADDR_SEQ); % Number of values to read

% Define the index data type based on the number of values
NT_ADDR_IDX = numerictype(false,ceil(log2(NUM_VALS))+1,0); % index

% State machine defines
STATE_IDLE = fi(0,NT_STATE,FM);           
STATE_ADDR = fi(1,NT_STATE,FM);
STATE_EN = fi(2,NT_STATE,FM);
STATE_WAIT = fi(3,NT_STATE,FM);
           
% Declare registers
persistent state val addr den addr_idx;

% Set reset values
if isempty(state)
    state = STATE_IDLE;
    val = fi(zeros(NUM_VALS,1),NT_VAL,FM);
    addr = fi(0,NT_ADDR,FM);
    den = false;
    addr_idx = fi(0,NT_ADDR_IDX,FM);
end

%% Drive the outputs
daddr_o = addr;
den_o = den;
val_o = val;

%% Control the state
switch (state)
    case STATE_IDLE
        % IDLE state, increment the index
        if (addr_idx == NUM_VALS)
            addr_idx(:) = 1;
        else
            addr_idx(:) = addr_idx + 1;
        end
        state(:) = STATE_ADDR;
    case STATE_ADDR
        % ADDR state, write out the address
        addr(:) = ADDR_SEQ(addr_idx);
        den(:) = false;
        state(:) = STATE_EN;
    case STATE_EN
        % EN state, drive the enable high
        state(:) = STATE_WAIT;
        den(:) = true;
    case STATE_WAIT
        % WAIT state, wait for drdy
        if (drdy_i)
            val(addr_idx) = do_i;
            state(:) = STATE_IDLE;
        end
        den(:) = false;
end
